simulink model "TST_PTODi_TrqDesCoord"  (R2016b)
settings: Solver=FixedStepDiscrete  StartTime=0.0  StopTime=simTime  FixedStep=sampleTime  RelTol=1e-3
values from neighbouring files (symbols this model uses):
  testCase = 1    [initTST_PTODi_TrqDesCoord_001.m]
libraries: simulink x6, UnitTest_Lib x4
settings Model: Creator=zhengjinyan  LastModifiedBy=zhengjinyan
settings DebuggingCC: SignalRangeChecking=error

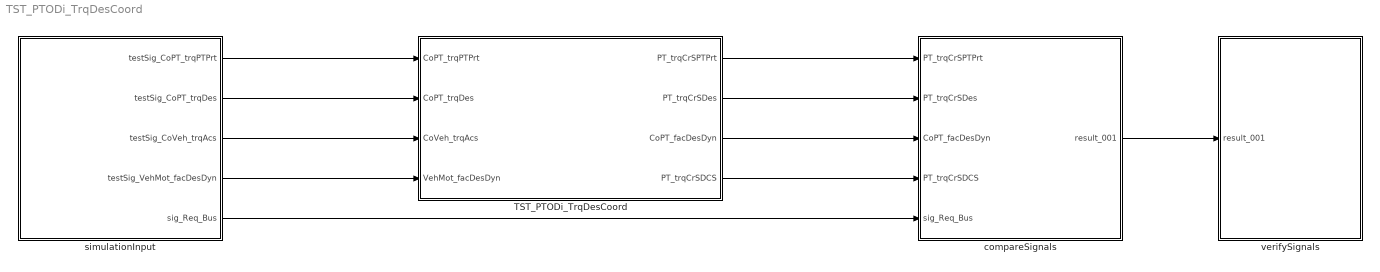
== system TST_PTODi_TrqDesCoord ==
  TST_PTODi_TrqDesCoord : Subsystem
  compareSignals : Subsystem
  simulationInput : Subsystem
  verifySignals : Subsystem
  wires:
  simulationInput/1(testSig_CoPT_trqPTPrt) -> TST_PTODi_TrqDesCoord/1(CoPT_trqPTPrt)
  simulationInput/2(testSig_CoPT_trqDes) -> TST_PTODi_TrqDesCoord/2(CoPT_trqDes)
  simulationInput/3(testSig_CoVeh_trqAcs) -> TST_PTODi_TrqDesCoord/3(CoVeh_trqAcs)
  simulationInput/4(testSig_VehMot_facDesDyn) -> TST_PTODi_TrqDesCoord/4(VehMot_facDesDyn)
  TST_PTODi_TrqDesCoord/1(PT_trqCrSPTPrt) -> compareSignals/1(PT_trqCrSPTPrt)
  TST_PTODi_TrqDesCoord/2(PT_trqCrSDes) -> compareSignals/2(PT_trqCrSDes)
  TST_PTODi_TrqDesCoord/3(CoPT_facDesDyn) -> compareSignals/3(CoPT_facDesDyn)
  TST_PTODi_TrqDesCoord/4(PT_trqCrSDCS) -> compareSignals/4(PT_trqCrSDCS)
  simulationInput/5(sig_Req_Bus) -> compareSignals/5(sig_Req_Bus)
  compareSignals/1(result_001) -> verifySignals/1(result_001)

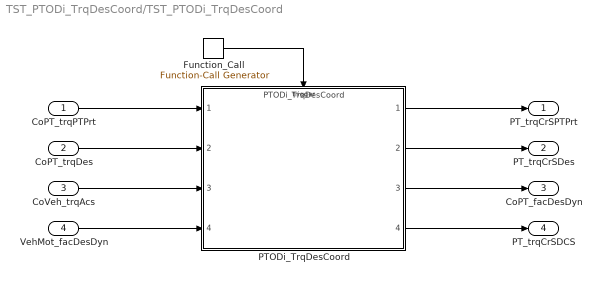
== system TST_PTODi_TrqDesCoord/TST_PTODi_TrqDesCoord ==
  CoPT_trqPTPrt : Inport
  CoPT_trqDes : Inport  Port=2
  CoVeh_trqAcs : Inport  Port=3
  VehMot_facDesDyn : Inport  Port=4
  Function_Call : simulink/Ports & Subsystems/Function-Call Generator  sample_time=sampleTime  numberOfIterations=1
  PTODi_TrqDesCoord : ModelReference  ModelNameDialog=PTODi_TrqDesCoord  SimulationMode=Normal  ModelReferenceVersion=1.8  TriggerPortName=function  TriggerPortTriggerType=function-call  TriggerPortStatesWhenEnabling=held
  PT_trqCrSPTPrt : Outport
  PT_trqCrSDes : Outport  Port=2
  CoPT_facDesDyn : Outport  Port=3
  PT_trqCrSDCS : Outport  Port=4
  wires:
  Function_Call/1 -> PTODi_TrqDesCoord/Trigger
  CoPT_trqPTPrt/1 -> PTODi_TrqDesCoord/1
  CoPT_trqDes/1 -> PTODi_TrqDesCoord/2
  CoVeh_trqAcs/1 -> PTODi_TrqDesCoord/3
  VehMot_facDesDyn/1 -> PTODi_TrqDesCoord/4
  PTODi_TrqDesCoord/1 -> PT_trqCrSPTPrt/1
  PTODi_TrqDesCoord/2 -> PT_trqCrSDes/1
  PTODi_TrqDesCoord/3 -> CoPT_facDesDyn/1
  PTODi_TrqDesCoord/4 -> PT_trqCrSDCS/1

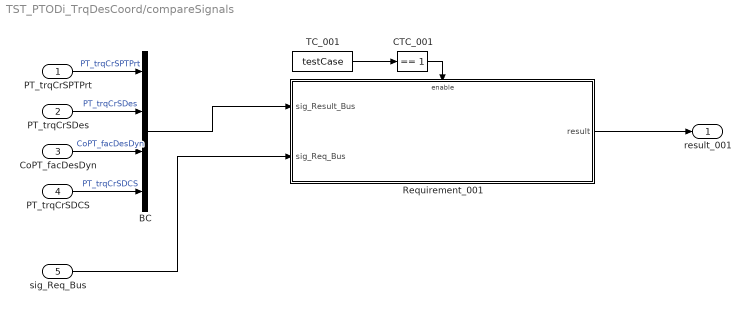
== system TST_PTODi_TrqDesCoord/compareSignals ==
  PT_trqCrSPTPrt : Inport
  PT_trqCrSDes : Inport  Port=2
  CoPT_facDesDyn : Inport  Port=3
  PT_trqCrSDCS : Inport  Port=4
  sig_Req_Bus : Inport  Port=5
  BC : BusCreator  Inputs=4
  CTC_001 : simulink/Logic and Bit Operations/Compare To Constant  relop===  const=1  OutDataTypeStr=boolean
  Requirement_001 : Subsystem
  TC_001 : Constant  Value=testCase
  result_001 : Outport
  wires:
  PT_trqCrSPTPrt/1 -> BC/1  "PT_trqCrSPTPrt"
  PT_trqCrSDes/1 -> BC/2  "PT_trqCrSDes"
  CoPT_facDesDyn/1 -> BC/3  "CoPT_facDesDyn"
  PT_trqCrSDCS/1 -> BC/4  "PT_trqCrSDCS"
  TC_001/1 -> CTC_001/1
  CTC_001/1 -> Requirement_001/Enable
  sig_Req_Bus/1 -> Requirement_001/2(sig_Req_Bus)
  BC/1 -> Requirement_001/1(sig_Result_Bus)
  Requirement_001/1(result) -> result_001/1

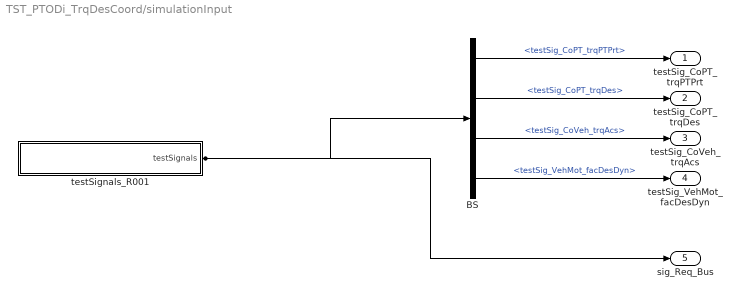
== system TST_PTODi_TrqDesCoord/simulationInput ==
  BS : BusSelector  OutputSignals=testSig_CoPT_trqPTPrt,testSig_CoPT_trqDes,testSig_CoVeh_trqAcs,testSig_VehMot_facDesDyn
  testSignals_R001 : Subsystem
  testSig_CoPT_trqPTPrt : Outport
  testSig_CoPT_trqDes : Outport  Port=2
  testSig_CoVeh_trqAcs : Outport  Port=3
  testSig_VehMot_facDesDyn : Outport  Port=4
  sig_Req_Bus : Outport  Port=5
  wires:
  BS/1 -> testSig_CoPT_trqPTPrt/1  "<testSig_CoPT_trqPTPrt>"
  BS/2 -> testSig_CoPT_trqDes/1  "<testSig_CoPT_trqDes>"
  BS/3 -> testSig_CoVeh_trqAcs/1  "<testSig_CoVeh_trqAcs>"
  BS/4 -> testSig_VehMot_facDesDyn/1  "<testSig_VehMot_facDesDyn>"
  testSignals_R001/1(testSignals) -> BS/1, sig_Req_Bus/1

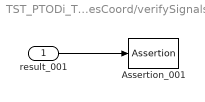
== system TST_PTODi_TrqDesCoord/verifySignals ==
  result_001 : Inport
  Assertion_001 : Assertion  Enabled=off
  wires:
  result_001/1 -> Assertion_001/1

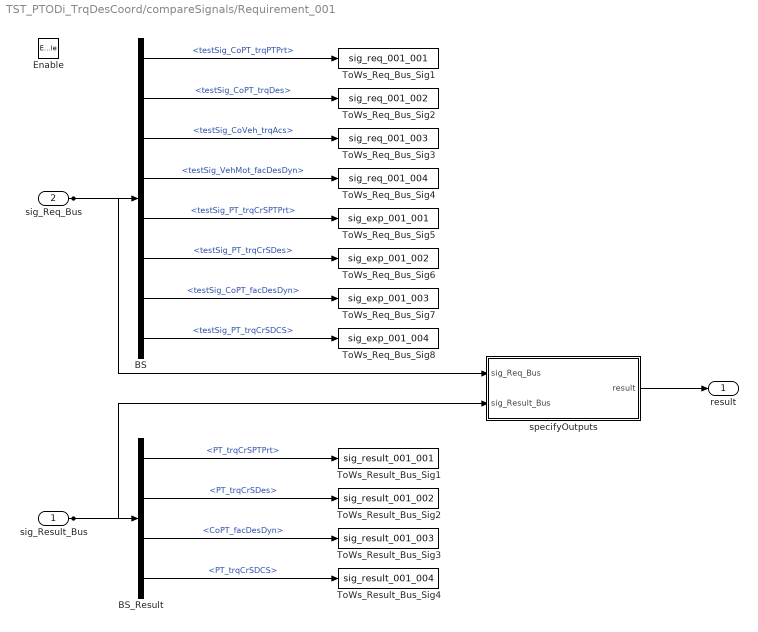
== system TST_PTODi_TrqDesCoord/compareSignals/Requirement_001 ==
  sig_Result_Bus : Inport
  sig_Req_Bus : Inport  Port=2
  Enable : EnablePort
  BS : BusSelector  OutputSignals=testSig_CoPT_trqPTPrt,testSig_CoPT_trqDes,testSig_CoVeh_trqAcs,testSig_VehMot_facDesDyn,testSig_PT_trqCrSPTPrt,testSig_PT_trqCrSDes,testSig_CoPT_facDesDyn,testSig_PT_trqCrSDCS
  BS_Result : BusSelector  OutputSignals=PT_trqCrSPTPrt,PT_trqCrSDes,CoPT_facDesDyn,PT_trqCrSDCS
  ToWs_Req_Bus_Sig1 : ToWorkspace  VariableName=sig_req_001_001  SaveFormat=Structure With Time
  ToWs_Req_Bus_Sig2 : ToWorkspace  VariableName=sig_req_001_002  SaveFormat=Structure With Time
  ToWs_Req_Bus_Sig3 : ToWorkspace  VariableName=sig_req_001_003  SaveFormat=Structure With Time
  ToWs_Req_Bus_Sig4 : ToWorkspace  VariableName=sig_req_001_004  SaveFormat=Structure With Time
  ToWs_Req_Bus_Sig5 : ToWorkspace  VariableName=sig_exp_001_001  SaveFormat=Structure With Time
  ToWs_Req_Bus_Sig6 : ToWorkspace  VariableName=sig_exp_001_002  SaveFormat=Structure With Time
  ToWs_Req_Bus_Sig7 : ToWorkspace  VariableName=sig_exp_001_003  SaveFormat=Structure With Time
  ToWs_Req_Bus_Sig8 : ToWorkspace  VariableName=sig_exp_001_004  SaveFormat=Structure With Time
  ToWs_Result_Bus_Sig1 : ToWorkspace  VariableName=sig_result_001_001  SaveFormat=Structure With Time
  ToWs_Result_Bus_Sig2 : ToWorkspace  VariableName=sig_result_001_002  SaveFormat=Structure With Time
  ToWs_Result_Bus_Sig3 : ToWorkspace  VariableName=sig_result_001_003  SaveFormat=Structure With Time
  ToWs_Result_Bus_Sig4 : ToWorkspace  VariableName=sig_result_001_004  SaveFormat=Structure With Time
  specifyOutputs : Subsystem
  result : Outport
  wires:
  sig_Req_Bus/1 -> BS/1, specifyOutputs/1(sig_Req_Bus)
  BS/1 -> ToWs_Req_Bus_Sig1/1  "<testSig_CoPT_trqPTPrt>"
  BS/2 -> ToWs_Req_Bus_Sig2/1  "<testSig_CoPT_trqDes>"
  BS/3 -> ToWs_Req_Bus_Sig3/1  "<testSig_CoVeh_trqAcs>"
  BS/4 -> ToWs_Req_Bus_Sig4/1  "<testSig_VehMot_facDesDyn>"
  BS/5 -> ToWs_Req_Bus_Sig5/1  "<testSig_PT_trqCrSPTPrt>"
  BS/6 -> ToWs_Req_Bus_Sig6/1  "<testSig_PT_trqCrSDes>"
  BS/7 -> ToWs_Req_Bus_Sig7/1  "<testSig_CoPT_facDesDyn>"
  BS/8 -> ToWs_Req_Bus_Sig8/1  "<testSig_PT_trqCrSDCS>"
  sig_Result_Bus/1 -> BS_Result/1, specifyOutputs/2(sig_Result_Bus)
  BS_Result/1 -> ToWs_Result_Bus_Sig1/1  "<PT_trqCrSPTPrt>"
  BS_Result/2 -> ToWs_Result_Bus_Sig2/1  "<PT_trqCrSDes>"
  BS_Result/3 -> ToWs_Result_Bus_Sig3/1  "<CoPT_facDesDyn>"
  BS_Result/4 -> ToWs_Result_Bus_Sig4/1  "<PT_trqCrSDCS>"
  specifyOutputs/1(result) -> result/1

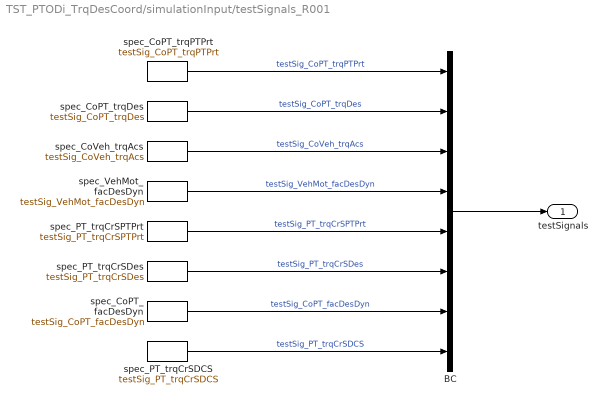
== system TST_PTODi_TrqDesCoord/simulationInput/testSignals_R001 ==
  BC : BusCreator  Inputs=8
  spec_CoPT_facDesDyn : FromWorkspace  VariableName=testSig_CoPT_facDesDyn  Interpolate=off  OutputAfterFinalValue=Holding final value
  spec_CoPT_trqDes : FromWorkspace  VariableName=testSig_CoPT_trqDes  Interpolate=off  OutputAfterFinalValue=Holding final value
  spec_CoPT_trqPTPrt : FromWorkspace  VariableName=testSig_CoPT_trqPTPrt  Interpolate=off  OutputAfterFinalValue=Holding final value
  spec_CoVeh_trqAcs : FromWorkspace  VariableName=testSig_CoVeh_trqAcs  Interpolate=off  OutputAfterFinalValue=Holding final value
  spec_PT_trqCrSDCS : FromWorkspace  VariableName=testSig_PT_trqCrSDCS  Interpolate=off  OutputAfterFinalValue=Holding final value
  spec_PT_trqCrSDes : FromWorkspace  VariableName=testSig_PT_trqCrSDes  Interpolate=off  OutputAfterFinalValue=Holding final value
  spec_PT_trqCrSPTPrt : FromWorkspace  VariableName=testSig_PT_trqCrSPTPrt  Interpolate=off  OutputAfterFinalValue=Holding final value
  spec_VehMot_facDesDyn : FromWorkspace  VariableName=testSig_VehMot_facDesDyn  Interpolate=off  OutputAfterFinalValue=Holding final value
  testSignals : Outport
  wires:
  BC/1 -> testSignals/1
  spec_CoPT_trqPTPrt/1 -> BC/1  "testSig_CoPT_trqPTPrt"
  spec_CoPT_trqDes/1 -> BC/2  "testSig_CoPT_trqDes"
  spec_CoVeh_trqAcs/1 -> BC/3  "testSig_CoVeh_trqAcs"
  spec_VehMot_facDesDyn/1 -> BC/4  "testSig_VehMot_facDesDyn"
  spec_PT_trqCrSPTPrt/1 -> BC/5  "testSig_PT_trqCrSPTPrt"
  spec_PT_trqCrSDes/1 -> BC/6  "testSig_PT_trqCrSDes"
  spec_CoPT_facDesDyn/1 -> BC/7  "testSig_CoPT_facDesDyn"
  spec_PT_trqCrSDCS/1 -> BC/8  "testSig_PT_trqCrSDCS"

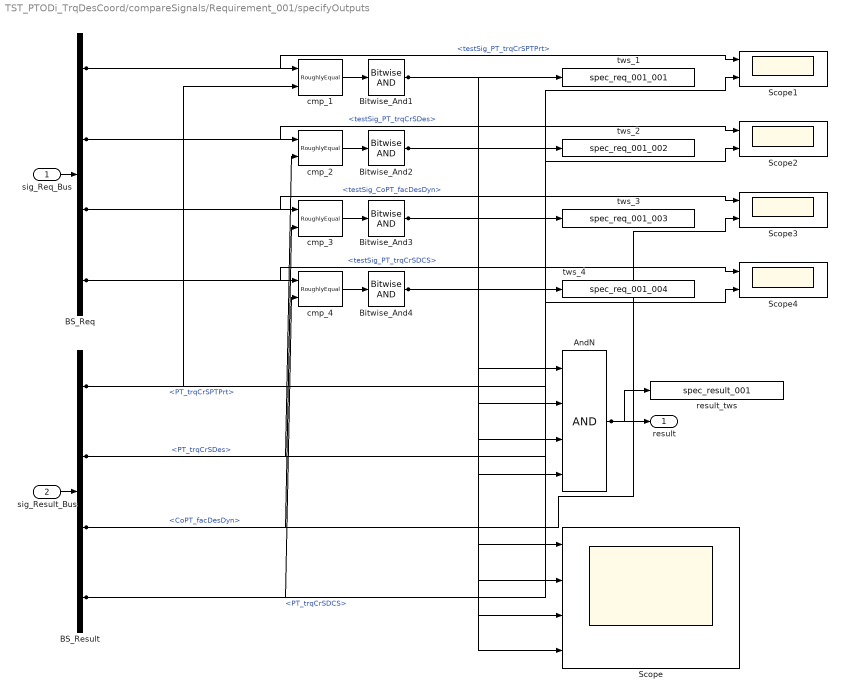
== system TST_PTODi_TrqDesCoord/compareSignals/Requirement_001/specifyOutputs ==
  sig_Req_Bus : Inport
  sig_Result_Bus : Inport  Port=2
  AndN : Logic  Inputs=4
  BS_Req : BusSelector  OutputSignals=testSig_PT_trqCrSPTPrt,testSig_PT_trqCrSDes,testSig_CoPT_facDesDyn,testSig_PT_trqCrSDCS
  BS_Result : BusSelector  OutputSignals=PT_trqCrSPTPrt,PT_trqCrSDes,CoPT_facDesDyn,PT_trqCrSDCS
  Bitwise_And{1..4} (4 alike) : simulink/Logic and Bit Operations/Bitwise Operator  logicop=AND  UseBitMask=off  BitMask=bin2dec('11011001')  BitMaskRealWorld=Stored Integer
  Scope : Scope  NumInputPorts=4
  Scope{1..4} (4 alike) : Scope  NumInputPorts=2
  cmp_{1..4} (4 alike) : UnitTest_Lib/RoughlyEqual  slope=0.1
  result_tws : ToWorkspace  VariableName=spec_result_001
  tws_1 : ToWorkspace  VariableName=spec_req_001_001
  tws_2 : ToWorkspace  VariableName=spec_req_001_002
  tws_3 : ToWorkspace  VariableName=spec_req_001_003
  tws_4 : ToWorkspace  VariableName=spec_req_001_004
  result : Outport
  wires:
  sig_Req_Bus/1 -> BS_Req/1
  sig_Result_Bus/1 -> BS_Result/1
  AndN/1 -> result/1, result_tws/1
  BS_Req/1 -> cmp_1/1, Scope1/1  "<testSig_PT_trqCrSPTPrt>"
  BS_Result/1 -> cmp_1/2, Scope1/2  "<PT_trqCrSPTPrt>"
  cmp_1/1 -> Bitwise_And1/1
  Bitwise_And1/1 -> tws_1/1, AndN/1, Scope/1
  BS_Req/2 -> cmp_2/1, Scope2/1  "<testSig_PT_trqCrSDes>"
  BS_Result/2 -> cmp_2/2, Scope2/2  "<PT_trqCrSDes>"
  cmp_2/1 -> Bitwise_And2/1
  Bitwise_And2/1 -> tws_2/1, AndN/2, Scope/2
  BS_Req/3 -> cmp_3/1, Scope3/1  "<testSig_CoPT_facDesDyn>"
  BS_Result/3 -> cmp_3/2, Scope3/2  "<CoPT_facDesDyn>"
  cmp_3/1 -> Bitwise_And3/1
  Bitwise_And3/1 -> tws_3/1, AndN/3, Scope/3
  BS_Req/4 -> cmp_4/1, Scope4/1  "<testSig_PT_trqCrSDCS>"
  BS_Result/4 -> cmp_4/2, Scope4/2  "<PT_trqCrSDCS>"
  cmp_4/1 -> Bitwise_And4/1
  Bitwise_And4/1 -> tws_4/1, AndN/4, Scope/4
